simulink model "wind_turbine_PID"  (Simulink 7.8)
settings: Solver=ode45  StartTime=0.0  StopTime=inf  RelTol=1e-3
values from neighbouring files (symbols this model uses):
  q = [x2;y2;c2;x3;y3;z3;a3;b3;c3;x4;y4;z4;b4;c4;x5;y5;z5;b5;c5;a6;b6;c6;a7;xSun;ySun;zSun;bSun;cSun;xPla1;yPla1;zPla1;bPla1;cPla1;xPla2;yPla2;zPla2;bPla2;cPla2;xPla3;yPla3;zPla3;bPla3;cPla3;xSecSt;ySecSt;zSecSt;bSecSt;cSecSt;a4;a5;aSun;aPla1;aPla2;aPla3;aSecSt;]    [environment.m]
libraries: simulink x1
settings Model: Creator=imac  LastModifiedBy=aitor
settings DebuggingCC: DiscreteInheritContinuousMsg=none  FcnCallInpInsideContextMsg=Use local settings

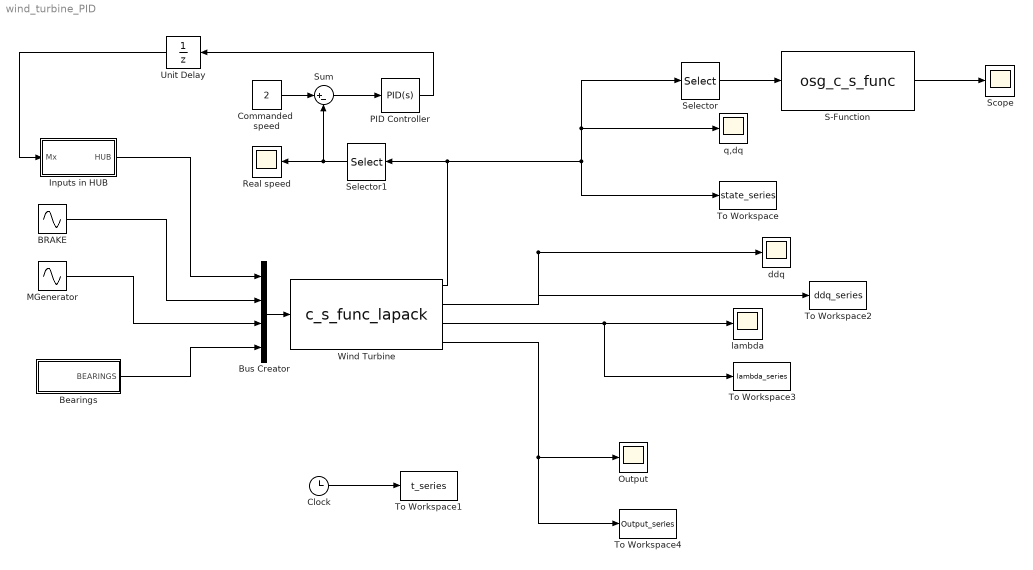
== system wind_turbine_PID ==
  BRAKE : Sin  Amplitude=0  Frequency=0  Phase=pi/2  SampleTime=0
  Bearings : Subsystem
  Bus Creator : BusCreator
  Clock : Clock
  Commanded  speed : Constant  Value=2
  Inputs in HUB : Subsystem
  MGenerator : Sin  Amplitude=0  Frequency=0  Phase=pi/2  SampleTime=0
  Output : Scope
      settings: YMin=0  YMax=170  SaveName=ScopeData3  SampleInput=on  SampleTime=0.01
  PID Controller : simulink/Continuous/PID Controller  Controller=PID  TimeDomain=Continuous-time  SampleTime=1  IntegratorMethod=Forward Euler  FilterMethod=Forward Euler  Form=Parallel  P=250  I=0  D=1  N=0  InitialConditionSource=internal  InitialConditionForIntegrator=0  InitialConditionForFilter=0  ExternalReset=none  LimitOutput=off  UpperSaturationLimit=inf  LowerSaturationLimit=-inf  LinearizeAsGain=off  AntiWindupMode=none  Kb=1  TrackingMode=off  Kt=1  PParamMin=[]  PParamMax=[]  IParamMin=[]  IParamMax=[]  DParamMin=[]  DParamMax=[]  NParamMin=[]  NParamMax=[]  KbParamMin=[]  KbParamMax=[]  KtParamMin=[]  KtParamMax=[]  POutMin=[]  POutMax=[]  IOutMin=[]  IOutMax=[]  DOutMin=[]  DOutMax=[]  NOutMin=[]  NOutMax=[]  KbOutMin=[]  KbOutMax=[]  KtOutMin=[]  KtOutMax=[]  IntegratorOutMin=[]  IntegratorOutMax=[]  FilterOutMin=[]  FilterOutMax=[]  SumOutMin=[]  SumOutMax=[]  SumI1OutMin=[]  SumI1OutMax=[]  SumI2OutMin=[]  SumI2OutMax=[]  SumI3OutMin=[]  SumI3OutMax=[]  SumDOutMin=[]  SumDOutMax=[]  SaturationOutMin=[]  SaturationOutMax=[]  IntegratorContinuousStateAttributes=''  IntegratorStateMustResolveToSignalObject=off  IntegratorRTWStateStorageClass=Auto  FilterContinuousStateAttributes=''  FilterStateMustResolveToSignalObject=off  FilterRTWStateStorageClass=Auto
  Real speed : Scope
      settings: TimeRange=10  YMin=0.0325  YMax=0.0575  SaveName=ScopeData5
  S-Function : S-Function  FunctionName=osg_c_s_func  EnableBusSupport=off
  Scope : Scope
      settings: YMin=-0.0001  YMax=6e-05  SaveName=ScopeData4
  Selector : Selector  InputPortWidth=2*length(q)  IndexOptions=Index vector (dialog)  Indices=1:1:length(q)  OutputSizes=1
  Selector1 : Selector  InputPortWidth=2*length(q)  IndexOptions=Index vector (dialog)  Indices=length(q)+7  OutputSizes=1
  Sum : Sum  Inputs=|+-
  To Workspace : ToWorkspace  VariableName=state_series  SampleTime=0.01  SaveFormat=Array
  To Workspace1 : ToWorkspace  VariableName=t_series  SampleTime=0.01  SaveFormat=Array
  To Workspace2 : ToWorkspace  VariableName=ddq_series  SampleTime=0.01  SaveFormat=Array
  To Workspace3 : ToWorkspace  VariableName=lambda_series  SampleTime=0.01  SaveFormat=Array
  To Workspace4 : ToWorkspace  VariableName=Output_series  SampleTime=0.01  SaveFormat=Array
  Unit Delay : UnitDelay  SampleTime=-1
  Wind Turbine : S-Function  FunctionName=c_s_func_lapack  Parameters=q dq param  EnableBusSupport=off
      mask Type: S-function: mycsfunc
      mask Description: This is a S-function that does the continuous state space system.
      mask Display: disp('[M , Phi_q''] [ddq]\n[Phi_q , 0] [lambda]\n=\n [Q ] \n   [gamma] ');
  ddq : Scope
      settings: YMin=-500  YMax=300  SampleInput=on  SampleTime=0.01
  lambda : Scope
      settings: YMin=-1750  YMax=1000  SaveName=ScopeData2  SampleInput=on  SampleTime=0.01
  q,dq : Scope
      settings: YMin=-2  YMax=7.5  SampleInput=on  SampleTime=0.01
  wires:
  Clock/1 -> To Workspace1/1
  Wind Turbine/1 -> Selector1/1, To Workspace/1, q,dq/1, Selector/1
  Wind Turbine/2 -> ddq/1, To Workspace2/1
  Wind Turbine/3 -> lambda/1, To Workspace3/1
  Wind Turbine/4 -> Output/1, To Workspace4/1
  Selector/1 -> S-Function/1
  S-Function/1 -> Scope/1
  Inputs in HUB/1(HUB) -> Bus Creator/1
  Bus Creator/1 -> Wind Turbine/1
  BRAKE/1 -> Bus Creator/2
  MGenerator/1 -> Bus Creator/3
  Bearings/1(BEARINGS) -> Bus Creator/4
  Selector1/1 -> Sum/2, Real speed/1
  Commanded  speed/1 -> Sum/1
  Sum/1 -> PID Controller/1
  PID Controller/1 -> Unit Delay/1
  Unit Delay/1 -> Inputs in HUB/1(Mx)

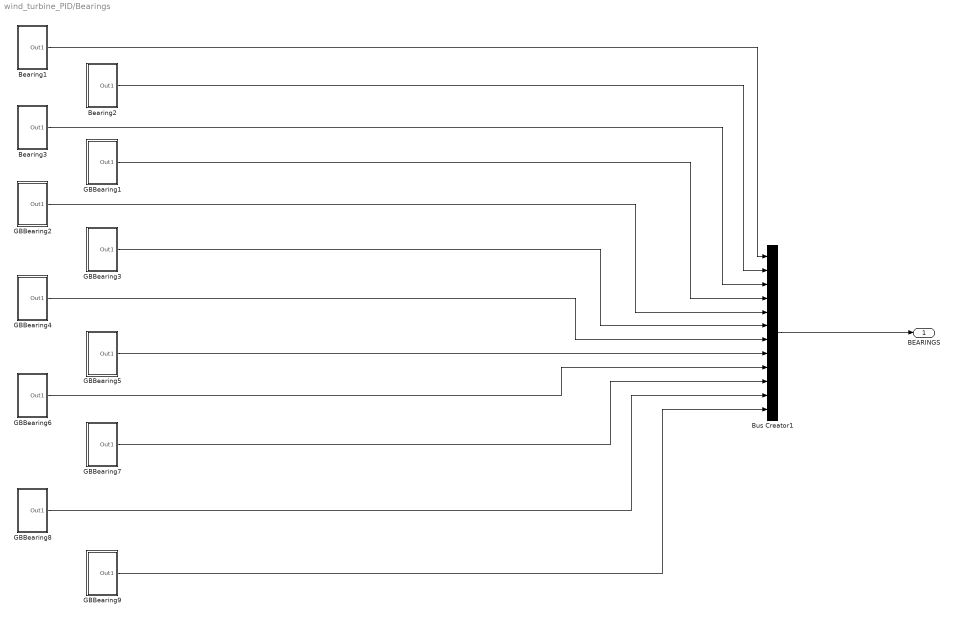
== system wind_turbine_PID/Bearings ==
  " GBBearing2" : Subsystem
  Bearing1 : Subsystem
  Bearing2 : Subsystem
  Bearing3 : Subsystem
  Bus Creator1 : BusCreator  Inputs=12
  GBBearing1 : Subsystem
  GBBearing3 : Subsystem
  GBBearing4 : Subsystem
  GBBearing5 : Subsystem
  GBBearing6 : Subsystem
  GBBearing7 : Subsystem
  GBBearing8 : Subsystem
  GBBearing9 : Subsystem
  BEARINGS : Outport
  wires:
  Bearing1/1(Out1) -> Bus Creator1/1
  Bearing2/1(Out1) -> Bus Creator1/2
  Bearing3/1(Out1) -> Bus Creator1/3
  GBBearing1/1(Out1) -> Bus Creator1/4
  Bus Creator1/1 -> BEARINGS/1
  " GBBearing2"/1(Out1) -> Bus Creator1/5
  GBBearing3/1(Out1) -> Bus Creator1/6
  GBBearing4/1(Out1) -> Bus Creator1/7
  GBBearing5/1(Out1) -> Bus Creator1/8
  GBBearing6/1(Out1) -> Bus Creator1/9
  GBBearing7/1(Out1) -> Bus Creator1/10
  GBBearing8/1(Out1) -> Bus Creator1/11
  GBBearing9/1(Out1) -> Bus Creator1/12

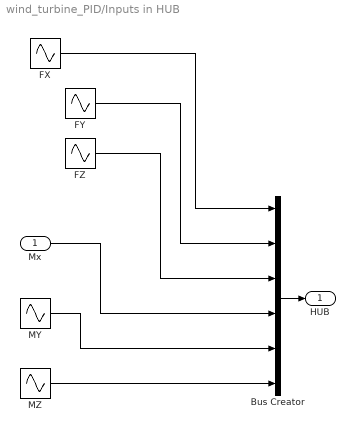
== system wind_turbine_PID/Inputs in HUB ==
  Mx : Inport
  Bus Creator : BusCreator  Inputs=6
  FX : Sin  Description=FX  Amplitude=0  Frequency=0  Phase=pi/2  SampleTime=0
  FY : Sin  Amplitude=0  Frequency=0  Phase=pi/2  SampleTime=0
  FZ : Sin  Amplitude=0  Frequency=0  Phase=pi/2  SampleTime=0
  MY : Sin  Amplitude=0  Frequency=0  Phase=pi/2  SampleTime=0
  MZ : Sin  Amplitude=0  Frequency=0  Phase=pi/2  SampleTime=0
  HUB : Outport
  wires:
  FX/1 -> Bus Creator/1
  FY/1 -> Bus Creator/2
  Mx/1 -> Bus Creator/4
  MY/1 -> Bus Creator/5
  MZ/1 -> Bus Creator/6
  FZ/1 -> Bus Creator/3
  Bus Creator/1 -> HUB/1

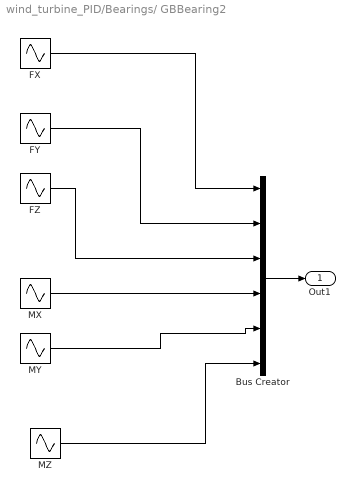
== system wind_turbine_PID/Bearings/ GBBearing2 ==
  Bus Creator : BusCreator  Inputs=6
  FX : Sin  Description=FX  Amplitude=0  Frequency=0  Phase=pi/2  SampleTime=0
  FY : Sin  Amplitude=0  Frequency=0  Phase=pi/2  SampleTime=0
  FZ : Sin  Amplitude=0  Frequency=0  Phase=pi/2  SampleTime=0
  MX : Sin  Amplitude=0  Frequency=0  Phase=pi/2  SampleTime=0
  MY : Sin  Amplitude=0  Frequency=0  Phase=pi/2  SampleTime=0
  MZ : Sin  Amplitude=0  Frequency=0  Phase=pi/2  SampleTime=0
  Out1 : Outport
  wires:
  FX/1 -> Bus Creator/1
  FY/1 -> Bus Creator/2
  MX/1 -> Bus Creator/4
  MY/1 -> Bus Creator/5
  MZ/1 -> Bus Creator/6
  FZ/1 -> Bus Creator/3
  Bus Creator/1 -> Out1/1

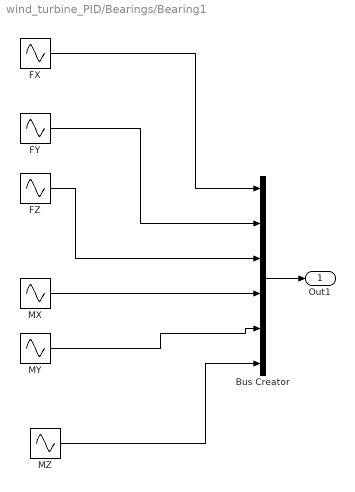
== system wind_turbine_PID/Bearings/Bearing1 ==
  Bus Creator : BusCreator  Inputs=6
  FX : Sin  Description=FX  Amplitude=0  Frequency=0  Phase=pi/2  SampleTime=0
  FY : Sin  Amplitude=0  Frequency=0  Phase=pi/2  SampleTime=0
  FZ : Sin  Amplitude=0  Frequency=0  Phase=pi/2  SampleTime=0
  MX : Sin  Amplitude=0  Frequency=0  Phase=pi/2  SampleTime=0
  MY : Sin  Amplitude=0  Frequency=0  Phase=pi/2  SampleTime=0
  MZ : Sin  Amplitude=0  Frequency=0  Phase=pi/2  SampleTime=0
  Out1 : Outport
  wires:
  FX/1 -> Bus Creator/1
  FY/1 -> Bus Creator/2
  MX/1 -> Bus Creator/4
  MY/1 -> Bus Creator/5
  MZ/1 -> Bus Creator/6
  FZ/1 -> Bus Creator/3
  Bus Creator/1 -> Out1/1

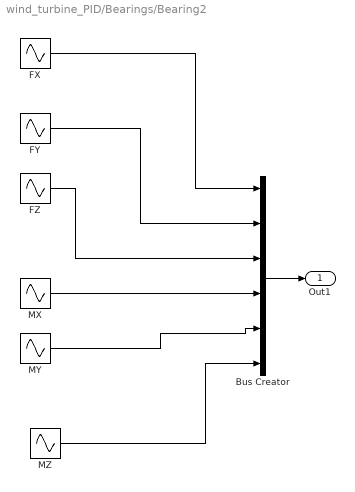
== system wind_turbine_PID/Bearings/Bearing2 ==
  Bus Creator : BusCreator  Inputs=6
  FX : Sin  Description=FX  Amplitude=0  Frequency=0  Phase=pi/2  SampleTime=0
  FY : Sin  Amplitude=0  Frequency=0  Phase=pi/2  SampleTime=0
  FZ : Sin  Amplitude=0  Frequency=pi/2  SampleTime=0
  MX : Sin  Amplitude=0  Frequency=0  Phase=pi/2  SampleTime=0
  MY : Sin  Amplitude=0  Frequency=0  Phase=pi/2  SampleTime=0
  MZ : Sin  Amplitude=0  Frequency=0  Phase=pi/2  SampleTime=0
  Out1 : Outport
  wires:
  FX/1 -> Bus Creator/1
  FY/1 -> Bus Creator/2
  MX/1 -> Bus Creator/4
  MY/1 -> Bus Creator/5
  MZ/1 -> Bus Creator/6
  FZ/1 -> Bus Creator/3
  Bus Creator/1 -> Out1/1

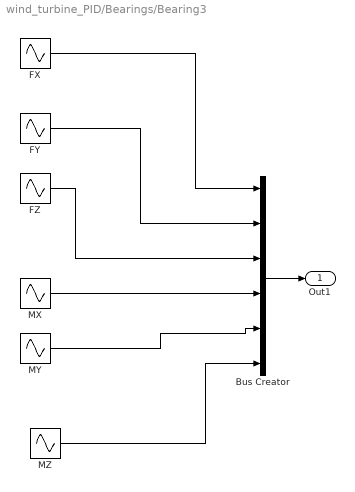
== system wind_turbine_PID/Bearings/Bearing3 ==
  Bus Creator : BusCreator  Inputs=6
  FX : Sin  Description=FX  Amplitude=0  Frequency=0  Phase=pi/2  SampleTime=0
  FY : Sin  Amplitude=0  Frequency=0  Phase=pi/2  SampleTime=0
  FZ : Sin  Amplitude=0  Frequency=0  Phase=pi/2  SampleTime=0
  MX : Sin  Amplitude=0  Frequency=0  Phase=pi/2  SampleTime=0
  MY : Sin  Amplitude=0  Frequency=0  Phase=pi/2  SampleTime=0
  MZ : Sin  Amplitude=0  Frequency=0  Phase=pi/2  SampleTime=0
  Out1 : Outport
  wires:
  FX/1 -> Bus Creator/1
  FY/1 -> Bus Creator/2
  MX/1 -> Bus Creator/4
  MY/1 -> Bus Creator/5
  MZ/1 -> Bus Creator/6
  FZ/1 -> Bus Creator/3
  Bus Creator/1 -> Out1/1

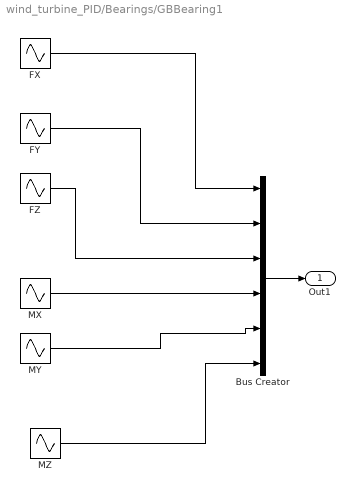
== system wind_turbine_PID/Bearings/GBBearing1 ==
  Bus Creator : BusCreator  Inputs=6
  FX : Sin  Description=FX  Amplitude=0  Frequency=0  Phase=pi/2  SampleTime=0
  FY : Sin  Amplitude=0  Frequency=0  Phase=pi/2  SampleTime=0
  FZ : Sin  Amplitude=0  Frequency=pi/2  SampleTime=0
  MX : Sin  Amplitude=0  Frequency=0  Phase=pi/2  SampleTime=0
  MY : Sin  Amplitude=0  Frequency=0  Phase=pi/2  SampleTime=0
  MZ : Sin  Amplitude=0  Frequency=0  Phase=pi/2  SampleTime=0
  Out1 : Outport
  wires:
  FX/1 -> Bus Creator/1
  FY/1 -> Bus Creator/2
  MX/1 -> Bus Creator/4
  MY/1 -> Bus Creator/5
  MZ/1 -> Bus Creator/6
  FZ/1 -> Bus Creator/3
  Bus Creator/1 -> Out1/1

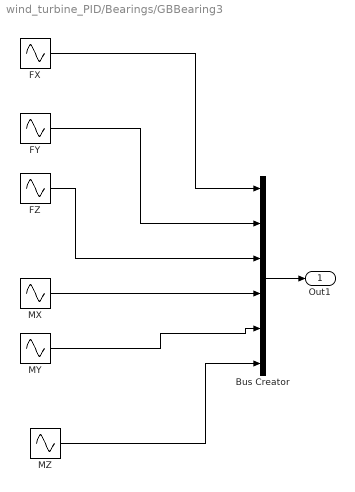
== system wind_turbine_PID/Bearings/GBBearing3 ==
  Bus Creator : BusCreator  Inputs=6
  FX : Sin  Description=FX  Amplitude=0  Frequency=0  Phase=pi/2  SampleTime=0
  FY : Sin  Amplitude=0  Frequency=0  Phase=pi/2  SampleTime=0
  FZ : Sin  Amplitude=0  Frequency=0  Phase=pi/2  SampleTime=0
  MX : Sin  Amplitude=0  Frequency=0  Phase=pi/2  SampleTime=0
  MY : Sin  Amplitude=0  Frequency=0  Phase=pi/2  SampleTime=0
  MZ : Sin  Amplitude=0  Frequency=0  Phase=pi/2  SampleTime=0
  Out1 : Outport
  wires:
  FX/1 -> Bus Creator/1
  FY/1 -> Bus Creator/2
  MX/1 -> Bus Creator/4
  MY/1 -> Bus Creator/5
  MZ/1 -> Bus Creator/6
  FZ/1 -> Bus Creator/3
  Bus Creator/1 -> Out1/1

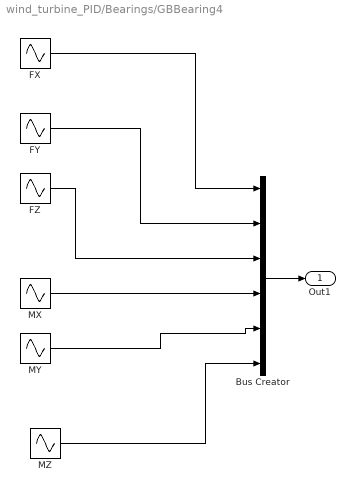
== system wind_turbine_PID/Bearings/GBBearing4 ==
  Bus Creator : BusCreator  Inputs=6
  FX : Sin  Description=FX  Amplitude=0  Frequency=0  Phase=pi/2  SampleTime=0
  FY : Sin  Amplitude=0  Frequency=0  Phase=pi/2  SampleTime=0
  FZ : Sin  Amplitude=0  Frequency=0  Phase=pi/2  SampleTime=0
  MX : Sin  Amplitude=0  Frequency=0  Phase=pi/2  SampleTime=0
  MY : Sin  Amplitude=0  Frequency=0  Phase=pi/2  SampleTime=0
  MZ : Sin  Amplitude=0  Frequency=0  Phase=pi/2  SampleTime=0
  Out1 : Outport
  wires:
  FX/1 -> Bus Creator/1
  FY/1 -> Bus Creator/2
  MX/1 -> Bus Creator/4
  MY/1 -> Bus Creator/5
  MZ/1 -> Bus Creator/6
  FZ/1 -> Bus Creator/3
  Bus Creator/1 -> Out1/1

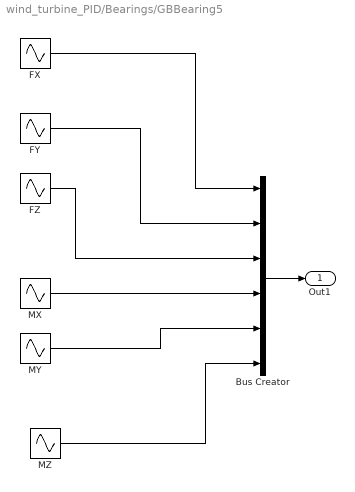
== system wind_turbine_PID/Bearings/GBBearing5 ==
  Bus Creator : BusCreator  Inputs=6
  FX : Sin  Description=FX  Amplitude=0  Frequency=0  Phase=pi/2  SampleTime=0
  FY : Sin  Amplitude=0  Frequency=0  Phase=pi/2  SampleTime=0
  FZ : Sin  Amplitude=0  Frequency=0  Phase=pi/2  SampleTime=0
  MX : Sin  Amplitude=0  Frequency=0  Phase=pi/2  SampleTime=0
  MY : Sin  Amplitude=0  Frequency=0  Phase=pi/2  SampleTime=0
  MZ : Sin  Amplitude=0  Frequency=0  Phase=pi/2  SampleTime=0
  Out1 : Outport
  wires:
  FX/1 -> Bus Creator/1
  FY/1 -> Bus Creator/2
  MX/1 -> Bus Creator/4
  MY/1 -> Bus Creator/5
  MZ/1 -> Bus Creator/6
  FZ/1 -> Bus Creator/3
  Bus Creator/1 -> Out1/1

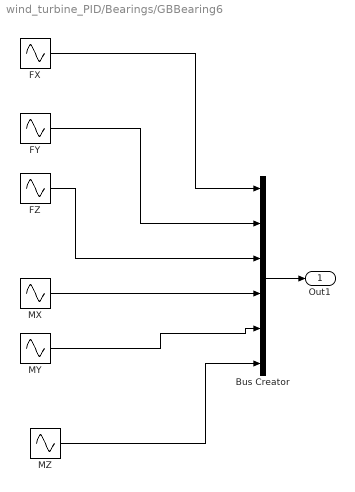
== system wind_turbine_PID/Bearings/GBBearing6 ==
  Bus Creator : BusCreator  Inputs=6
  FX : Sin  Description=FX  Amplitude=0  Frequency=0  Phase=pi/2  SampleTime=0
  FY : Sin  Amplitude=0  Frequency=0  Phase=pi/2  SampleTime=0
  FZ : Sin  Amplitude=0  Frequency=0  Phase=pi/2  SampleTime=0
  MX : Sin  Amplitude=0  Frequency=0  Phase=pi/2  SampleTime=0
  MY : Sin  Amplitude=0  Frequency=0  Phase=pi/2  SampleTime=0
  MZ : Sin  Amplitude=0  Frequency=0  Phase=pi/2  SampleTime=0
  Out1 : Outport
  wires:
  FX/1 -> Bus Creator/1
  FY/1 -> Bus Creator/2
  MX/1 -> Bus Creator/4
  MY/1 -> Bus Creator/5
  MZ/1 -> Bus Creator/6
  FZ/1 -> Bus Creator/3
  Bus Creator/1 -> Out1/1

== system wind_turbine_PID/Bearings/GBBearing7 ==
  Bus Creator : BusCreator  Inputs=6
  FX : Sin  Description=FX  Amplitude=0  Frequency=0  Phase=pi/2  SampleTime=0
  FY : Sin  Amplitude=0  Frequency=0  Phase=pi/2  SampleTime=0
  FZ : Sin  Amplitude=0  Frequency=100  Phase=pi/2  SampleTime=0
  MX : Sin  Amplitude=0  Frequency=0  Phase=pi/2  SampleTime=0
  MY : Sin  Amplitude=0  Frequency=0  Phase=pi/2  SampleTime=0
  MZ : Sin  Amplitude=0  Frequency=0  Phase=pi/2  SampleTime=0
  Out1 : Outport
  wires:
  FX/1 -> Bus Creator/1
  FY/1 -> Bus Creator/2
  MX/1 -> Bus Creator/4
  MY/1 -> Bus Creator/5
  MZ/1 -> Bus Creator/6
  FZ/1 -> Bus Creator/3
  Bus Creator/1 -> Out1/1

== system wind_turbine_PID/Bearings/GBBearing8 ==
  Bus Creator : BusCreator  Inputs=6
  FX : Sin  Description=FX  Amplitude=0  Frequency=0  Phase=pi/2  SampleTime=0
  FY : Sin  Amplitude=0  Frequency=0  Phase=pi/2  SampleTime=0
  FZ : Sin  Amplitude=0  Frequency=100  Phase=pi/2  SampleTime=0
  MX : Sin  Amplitude=0  Frequency=0  Phase=pi/2  SampleTime=0
  MY : Sin  Amplitude=0  Frequency=0  Phase=pi/2  SampleTime=0
  MZ : Sin  Amplitude=0  Frequency=0  Phase=pi/2  SampleTime=0
  Out1 : Outport
  wires:
  FX/1 -> Bus Creator/1
  FY/1 -> Bus Creator/2
  MX/1 -> Bus Creator/4
  MY/1 -> Bus Creator/5
  MZ/1 -> Bus Creator/6
  FZ/1 -> Bus Creator/3
  Bus Creator/1 -> Out1/1

== system wind_turbine_PID/Bearings/GBBearing9 ==
  Bus Creator : BusCreator  Inputs=6
  FX : Sin  Description=FX  Amplitude=0  Frequency=0  Phase=pi/2  SampleTime=0
  FY : Sin  Amplitude=0  Frequency=0  Phase=pi/2  SampleTime=0
  FZ : Sin  Amplitude=0  Frequency=0  Phase=pi/2  SampleTime=0
  MX : Sin  Amplitude=0  Frequency=0  Phase=pi/2  SampleTime=0
  MY : Sin  Amplitude=0  Frequency=0  Phase=pi/2  SampleTime=0
  MZ : Sin  Amplitude=0  Frequency=0  Phase=pi/2  SampleTime=0
  Out1 : Outport
  wires:
  FX/1 -> Bus Creator/1
  FY/1 -> Bus Creator/2
  MX/1 -> Bus Creator/4
  MY/1 -> Bus Creator/5
  MZ/1 -> Bus Creator/6
  FZ/1 -> Bus Creator/3
  Bus Creator/1 -> Out1/1
